simulink model "WaterHeater"  (R2015b)
settings: Solver=ode23s  SolverMode=SingleTasking  StartTime=0.0  StopTime=sim_time  RelTol=1e-3
model workspace (MAT data in the model file):
  actuation_delay = 1
  ambient_temp = 65
  ambient_temperature = 25
  final_ref_temp = 135
  initial_ref_temp = 65
  quantization_step = 0.5
  sensor_delay = 0.1
  simTime = 10
  step_time = 2
libraries: simulink x1
settings Model: Creator=jyotirmoy  LastModifiedBy=xjin
settings DataIOCC: SaveFormat=Array  SignalLoggingSaveFormat=ModelDataLogs
settings OptimizationCC: BlockReduction=off  BooleanDataType=off
settings DebuggingCC: SaveWithParameterizedLinksMsg=none  UnderspecifiedInitializationDetection=Classic  MergeDetectMultiDrivingBlocksExec=none  SignalResolutionControl=TryResolveAllWithWarning  MultiTaskDSMMsg=warning  MultiTaskCondExecSysMsg=none  StateNameClashWarn=warning
settings HardwareCC: ProdBitPerPointer=32  ProdLargestAtomicFloat=None  ProdIntDivRoundTo=Undefined  ProdEndianess=Unspecified  ProdWordSize=32  ProdHWDeviceType=32-bit Generic  TargetUnknown=on
settings GRTTargetCC: GeneratePreprocessorConditionals=Disable all
settings ConfigComp: CovModelRefEnable=Off

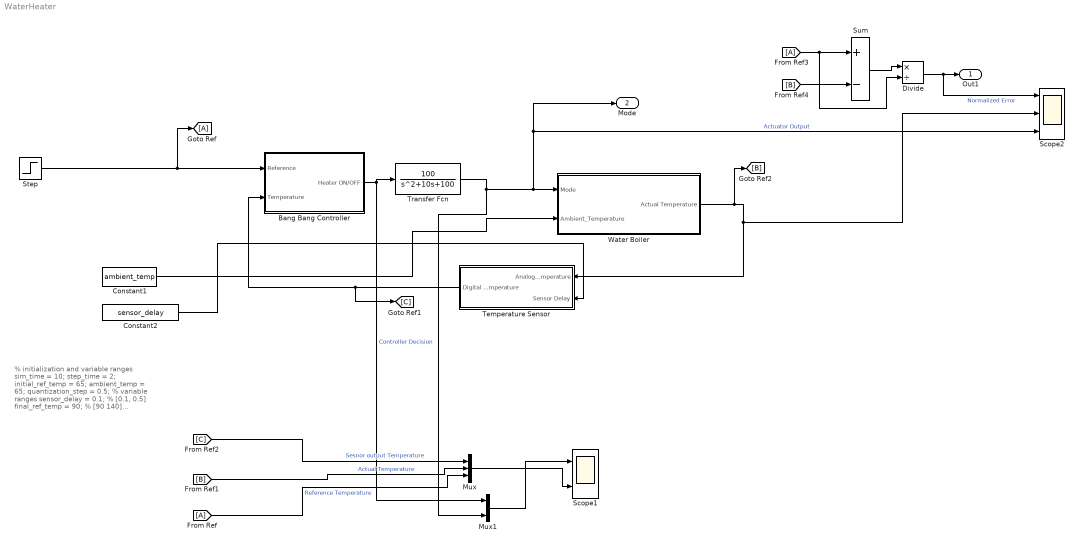
== system WaterHeater ==
  note: % initialization and variable ranges
      | sim_time = 10;
      | step_time = 2;
      | initial_ref_temp = 65;
      | ambient_temp = 65;
      | quantization_step = 0.5;
      |
      | % variable ranges
      | sensor_delay = 0.1; % [0.1, 0.5]
      | final_ref_temp = 90; % [90 140]
      | actuation_delay = 0.5; % [0.5 1]
  Bang Bang Controller : Subsystem
  Constant1 : Constant  Value=ambient_temp
  Constant2 : Constant  Value=sensor_delay
  Divide : Product  Inputs=*/
  Mux : Mux  Inputs=3
  Mux1 : Mux  Inputs=2
  Scope1 : Scope  NumInputPorts=2
  Scope2 : Scope  NumInputPorts=3
  Step : Step  Time=step_time  Before=initial_ref_temp  After=final_ref_temp  SampleTime=0
  Sum : Sum  Inputs=+-
  Temperature Sensor : Subsystem
  Transfer Fcn : TransferFcn  Numerator=[100]  Denominator=[1 10 100]
  Water Boiler : Subsystem
  Out1 : Outport
  Mode : Outport  Port=2
  wires:
  Step/1 -> Bang Bang Controller/1(Reference), [A]
  Constant1/1 -> Water Boiler/2(Ambient_Temperature)
  Water Boiler/1(Actual Temperature) -> [B], Scope2/2, Temperature Sensor/1(Analog Temperature)
  [A] -> Mux/3  "Reference Temperature"
  Bang Bang Controller/1(Heater ON/OFF) -> Transfer Fcn/1, Mux1/1  "Controller Decision"
  Transfer Fcn/1 -> Mux1/2, Mode/1, Scope2/3, Water Boiler/1(Mode)  "Actuator Output"
  Constant2/1 -> Temperature Sensor/2(Sensor Delay)
  Temperature Sensor/1(Digital Temperature) -> [C], Bang Bang Controller/2(Temperature)
  [B] -> Mux/2  "Actual Temperature"
  [C] -> Mux/1  "Sesnor output Temperature"
  Mux/1 -> Scope1/2
  Mux1/1 -> Scope1/1
  [A] -> Divide/2, Sum/1
  [B] -> Sum/2
  Sum/1 -> Divide/1
  Divide/1 -> Scope2/1, Out1/1  "Normalized Error"

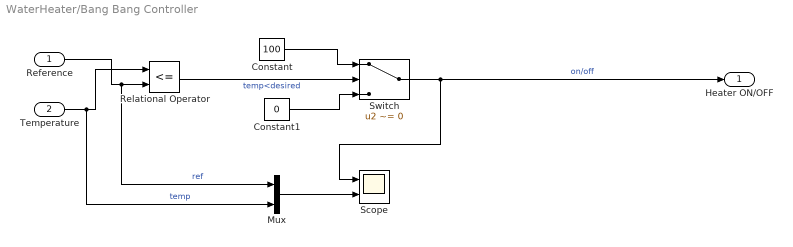
== system WaterHeater/Bang Bang Controller ==
  Reference : Inport
  Temperature : Inport  Port=2
  Constant : Constant  Value=100
  Constant1 : Constant  Value=0
  Mux : Mux  Inputs=2
  Relational Operator : RelationalOperator  Operator=<=  OutDataTypeStr=boolean
  Scope : Scope  NumInputPorts=2
  Switch : Switch  Criteria=u2 ~= 0
  Heater ON/OFF : Outport
  wires:
  Constant/1 -> Switch/1
  Constant1/1 -> Switch/3
  Reference/1 -> Mux/1, Relational Operator/2  "ref"
  Temperature/1 -> Mux/2, Relational Operator/1  "temp"
  Relational Operator/1 -> Switch/2  "temp<desired"
  Switch/1 -> Scope/1, Heater ON/OFF/1  "on/off"
  Mux/1 -> Scope/2

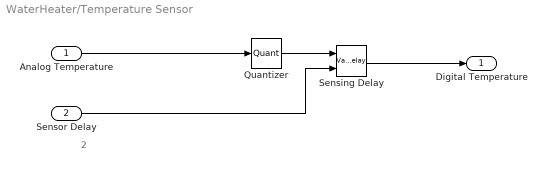
== system WaterHeater/Temperature Sensor ==
  note: 2
  Analog Temperature : Inport
  Sensor Delay : Inport  Port=2
  Quantizer : Quantizer  QuantizationInterval=quantization_step
  Sensing Delay : VariableTransportDelay  MaximumDelay=10
  Digital Temperature : Outport
  wires:
  Sensor Delay/1 -> Sensing Delay/2
  Sensing Delay/1 -> Digital Temperature/1
  Analog Temperature/1 -> Quantizer/1
  Quantizer/1 -> Sensing Delay/1

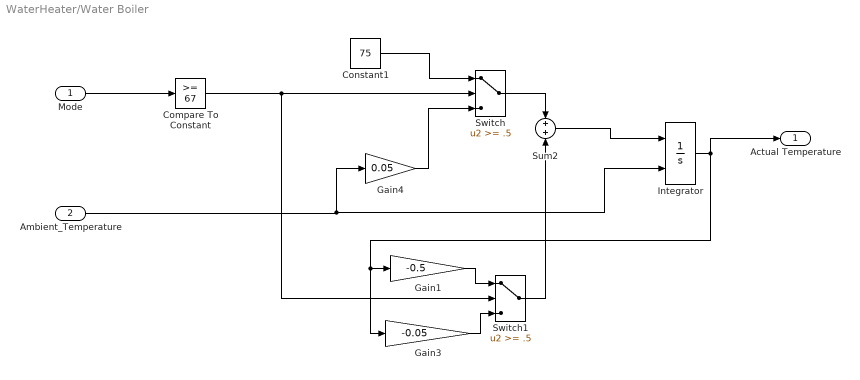
== system WaterHeater/Water Boiler ==
  Mode : Inport
  Ambient_Temperature : Inport  Port=2
  Compare To Constant : simulink/Logic and Bit Operations/Compare To Constant  relop=>=  const=67  OutDataTypeStr=boolean
  Constant1 : Constant  Value=75
  Gain1 : Gain  Gain=-0.5
  Gain3 : Gain  Gain=-0.05
  Gain4 : Gain  Gain=0.05
  Integrator : Integrator  InitialConditionSource=external  InitialCondition=20  ZeroCross=off
  Sum2 : Sum
  Switch : Switch  Threshold=.5  SaturateOnIntegerOverflow=on  InputSameDT=on
  Switch1 : Switch  Threshold=.5  SaturateOnIntegerOverflow=on  InputSameDT=on
  Actual Temperature : Outport
  wires:
  Compare To Constant/1 -> Switch1/2, Switch/2
  Mode/1 -> Compare To Constant/1
  Integrator/1 -> Actual Temperature/1, Gain3/1, Gain1/1
  Ambient_Temperature/1 -> Integrator/2, Gain4/1
  Constant1/1 -> Switch/1
  Switch/1 -> Sum2/1
  Switch1/1 -> Sum2/2
  Sum2/1 -> Integrator/1
  Gain3/1 -> Switch1/3
  Gain1/1 -> Switch1/1
  Gain4/1 -> Switch/3
